simulink model "ClosedLoop"  (R2016b)
settings: Solver=VariableStepAuto  StartTime=0.0  StopTime=30  RelTol=1e-3  EnableMultiTasking=on
values from neighbouring files (symbols this model uses):
  A = [0 0 1 0; 0 0 0 1; -k/J1 k/J1 -c/J1 c/J1; k/J2 -k/J2 c/J2 -c/J2]    [ELEC341Project.m]    (also in Question6and8.m)
  BI = [0; 0; kI/J1; 0]    [Question6and8.m]
  BTd = [0; 0; 0; 1/J2]    [Question6and8.m]
  C = [0 1 0 0]    [ELEC341Project.m]    (also in Question6and8.m)
  K = acker(A, B, CCLP)    [ELEC341Project.m]    (also in Question6and8.m = place(A, BI, CCLP))
  Kr = (-1 / (C*inv(A-B*K)*B))    [ELEC341Project.m]    (also in Question6and8.m = (-1 / (C*inv(A-BI*K)*BI)))
settings Model: PauseTimes=30  Creator=The MathWorks, Inc.  LastModifiedBy=isaacjacobsen
settings DataIOCC: LimitDataPoints=on
settings OptimizationCC: LifeSpan=inf
settings DebuggingCC: AllowSymbolicDim=off  SFUnexpectedBacktrackingDiag=warning  SFNoUnconditionalDefaultTransitionDiag=warning  SFExecutionAtInitializationDiag=none
settings ModelReferenceCC: PropagateSignalLabelsOutOfModel=off
settings GRTTargetCC: TargetLangStandard=C89/C90 (ANSI)
settings ConfigComp: CovMetricSettings=dw  CovHtmlReporting=on  CovSaveCumulativeToWorkspaceVar=on  CovSaveSingleToWorkspaceVar=on  CovExternalEMLEnable=off

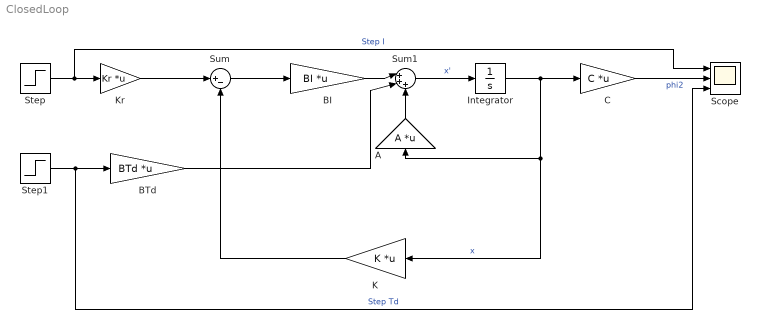
== system ClosedLoop ==
  A : Gain  Gain=A  Multiplication=Matrix(K*u)
  "BI " : Gain  Gain=BI  Multiplication=Matrix(K*u)
  BTd : Gain  Gain=BTd  Multiplication=Matrix(K*u)
  C : Gain  Gain=C  Multiplication=Matrix(K*u)
  Integrator : Integrator
  K : Gain  Gain=K  Multiplication=Matrix(K*u)
  Kr : Gain  Gain=Kr  Multiplication=Matrix(K*u)
  Scope : Scope  NumInputPorts=3
  Step : Step  Time=0  SampleTime=0.001
  Step1 : Step  Time=8  SampleTime=0.001
  Sum : Sum  Inputs=|+-
  Sum1 : Sum  Inputs=|+++
  wires:
  Step/1 -> Scope/1, Kr/1  "Step I"
  Kr/1 -> Sum/1
  Sum/1 -> "BI "/1
  "BI "/1 -> Sum1/1
  Sum1/1 -> Integrator/1  "x'"
  Integrator/1 -> A/1, K/1, C/1  "x"
  C/1 -> Scope/2  "phi2"
  K/1 -> Sum/2
  Step1/1 -> Scope/3, BTd/1  "Step Td"
  A/1 -> Sum1/3
  BTd/1 -> Sum1/2
